simulink model "simF16_u04"  (R2023b)
settings: Solver=ode4  StartTime=0  StopTime=5  FixedStep=0.005  RelTol=1e-3  EnableMultiTasking=on
values from neighbouring files (symbols this model uses):
  control_trim = u0    [find_trim.m]    (also in trimcond.mat = [0.154059600013 -0.694715670316 -3.42749873112e-15 4.5481145; trimcond2.mat = [0.154007747083 -0.694801754663 0.00182544197392 0.000329744)
  state_trim = constraint( state )    [find_trim.m]    (also in trimcond.mat = [502 0.0505701217863 2.65111802467e-16 0 0.0505701217863 0 0; trimcond2.mat = [501.999976668 0.0505473192089 -2.30406790676e-05 0.00010278)
settings Model: Creator=keviczky  LastModifiedBy=suvo
settings DataIOCC: Decimation=50  SaveFormat=Array  SignalLoggingSaveFormat=ModelDataLogs  ReturnWorkspaceOutputs=off  SignalLoggingName=sigsOut
settings OptimizationCC: BooleanDataType=off
settings DebuggingCC: SaveWithParameterizedLinksMsg=none  UnderspecifiedInitializationDetection=Classic  MergeDetectMultiDrivingBlocksExec=none  SignalResolutionControl=TryResolveAllWithWarning  MultiTaskDSMMsg=warning  MultiTaskCondExecSysMsg=none  UnconnectedInputMsg=warning  UnconnectedOutputMsg=warning  UnconnectedLineMsg=warning
settings HardwareCC: ProdBitPerPointer=32  ProdBitPerSizeT=32  ProdBitPerPtrDiffT=32  ProdLargestAtomicFloat=None  ProdIntDivRoundTo=Undefined  ProdEndianess=Unspecified  ProdWordSize=32  ProdHWDeviceType=32-bit Generic  TargetUnknown=on
settings ModelReferenceCC: PropagateSignalLabelsOutOfModel=off
settings GRTTargetCC: CombineOutputUpdateFcns=off  GRTInterface=on
settings ConfigComp: CovMetricSettings=dw  CovSaveCumulativeToWorkspaceVar=on  CovSaveSingleToWorkspaceVar=on

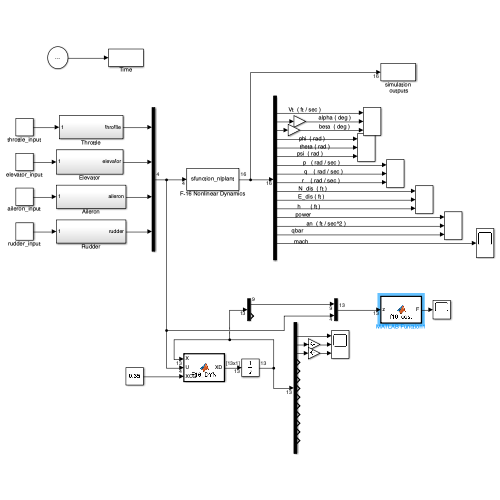
[thumbnail: Simulink's stored preview of the top-level diagram]
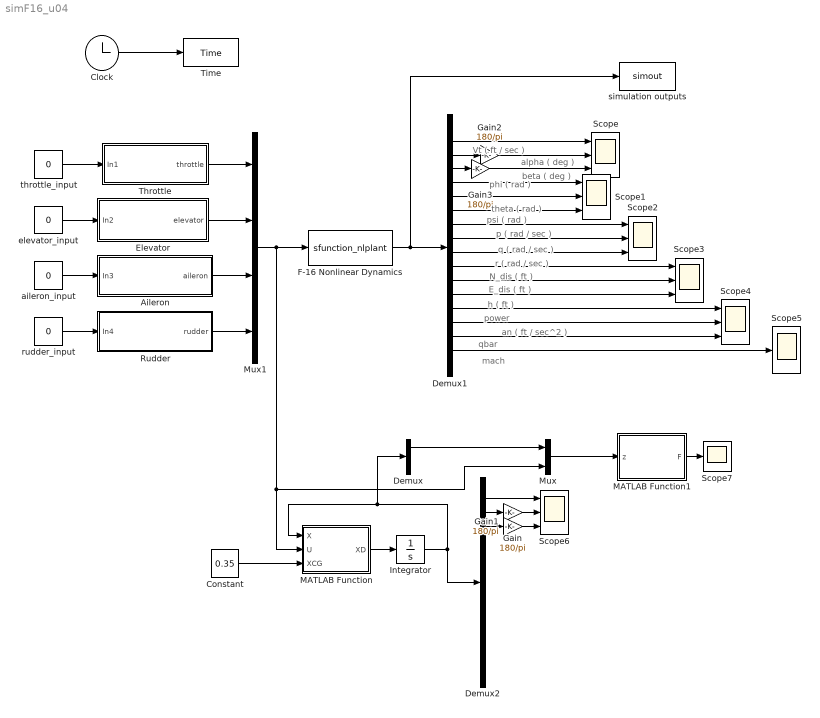
== system simF16_u04 ==
  note: Vt ( ft / sec )
  note: alpha ( deg )
  note: beta ( deg )
  note: phi ( rad )
  note: theta ( rad )
  note: psi ( rad )
  note: p ( rad / sec )
  note: q ( rad / sec )
  note: r ( rad / sec )
  note: N_dis ( ft )
  note: E_dis ( ft )
  note: h ( ft )
  note: power
  note: an ( ft / sec^2 )
  note: qbar
  note: mach
  Aileron : Subsystem
  Clock : Clock
      settings: Decimation=50
  Constant : Constant  Value=0.35
  Demux : Demux  Outputs=[9 4]
  Demux1 : Demux  Outputs=16
  Demux2 : Demux  Outputs=13
  Elevator : Subsystem
  F-16 Nonlinear Dynamics : S-Function  FunctionName=sfunction_nlplant  Parameters="state_trim,  xcg"  SFunctionDeploymentMode=off  EnableBusSupport=off
  Gain{,1..3} (4 alike) : Gain  Gain=180/pi
  Integrator : Integrator  InitialCondition=[state_trim]
  MATLAB Function : MATLAB Function  TreatAsAtomicUnit=on
  MATLAB Function1 : MATLAB Function  TreatAsAtomicUnit=on
  Mux : Mux  Inputs=2
  Mux1 : Mux
  Rudder : Subsystem
  Scope{,1..4,6} (6 alike) : Scope  NumInputPorts=3
  Scope5 : Scope
  Scope7 : Scope
  Throttle : Subsystem
  Time : ToWorkspace  VariableName=Time  SampleTime=-1
      settings: Decimation=100
  aileron_input : Constant  Value=0
  elevator_input : Constant  Value=0
  rudder_input : Constant  Value=0
  simulation outputs : ToWorkspace  VariableName=simout  SampleTime=-1
      settings: Decimation=100
  throttle_input : Constant  Value=0
  wires:
  F-16 Nonlinear Dynamics/1 -> Demux1/1, simulation outputs/1
  Clock/1 -> Time/1
  Demux1/1 -> Scope/1
  Demux1/2 -> Gain2/1
  Demux1/3 -> Gain3/1
  Demux1/5 -> Scope1/2
  Demux1/6 -> Scope1/3
  Demux1/7 -> Scope2/1
  Demux1/8 -> Scope2/2
  Demux1/9 -> Scope2/3
  Demux1/10 -> Scope3/1
  Demux1/11 -> Scope3/2
  Demux1/12 -> Scope3/3
  Demux1/13 -> Scope4/1
  Demux1/14 -> Scope4/2
  Demux1/4 -> Scope1/1
  Demux1/15 -> Scope4/3
  Demux1/16 -> Scope5/1
  Throttle/1(throttle) -> Mux1/1
  Elevator/1(elevator) -> Mux1/2
  Aileron/1(aileron) -> Mux1/3
  Rudder/1(rudder) -> Mux1/4
  throttle_input/1 -> Throttle/1(In1)
  elevator_input/1 -> Elevator/1(In2)
  aileron_input/1 -> Aileron/1(In3)
  rudder_input/1 -> Rudder/1(In4)
  MATLAB Function/1(XD) -> Integrator/1
  Integrator/1 -> Demux2/1, Demux/1, MATLAB Function/1(X)
  Mux1/1 -> MATLAB Function/2(U), Mux/2, F-16 Nonlinear Dynamics/1
  Demux2/1 -> Scope6/1
  Demux2/2 -> Gain/1
  Demux2/3 -> Gain1/1
  Constant/1 -> MATLAB Function/3(XCG)
  Gain/1 -> Scope6/2
  Gain1/1 -> Scope6/3
  Gain2/1 -> Scope/2
  Gain3/1 -> Scope/3
  MATLAB Function1/1(F) -> Scope7/1
  Demux/1 -> Mux/1
  Mux/1 -> MATLAB Function1/1(z)

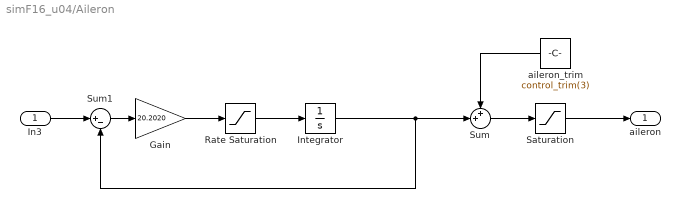
== system simF16_u04/Aileron ==
  In3 : Inport
  Gain : Gain  Gain=20.2020  SaturateOnIntegerOverflow=on  OutDataTypeStr=Inherit: Same as input  ParamDataTypeStr=Inherit: Same as input
  Integrator : Integrator  UpperSaturationLimit=21.5  LowerSaturationLimit=-21.5
  Rate Saturation : Saturate  UpperLimit=80  LowerLimit=-80
  Saturation : Saturate  UpperLimit=21.5  LowerLimit=-21.5
  Sum : Sum  Inputs=++|  InputSameDT=on  SaturateOnIntegerOverflow=on  OutDataTypeStr=Inherit: Same as first input
  Sum1 : Sum  Inputs=|+-  InputSameDT=on  SaturateOnIntegerOverflow=on  OutDataTypeStr=Inherit: Same as first input
  aileron_trim : Constant  Value=control_trim(3)
  aileron : Outport
  wires:
  In3/1 -> Sum1/1
  Sum1/1 -> Gain/1
  Gain/1 -> Rate Saturation/1
  Rate Saturation/1 -> Integrator/1
  Integrator/1 -> Sum1/2, Sum/2
  Sum/1 -> Saturation/1
  aileron_trim/1 -> Sum/1
  Saturation/1 -> aileron/1

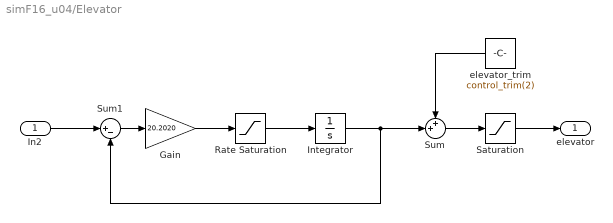
== system simF16_u04/Elevator ==
  In2 : Inport
  Gain : Gain  Gain=20.2020  SaturateOnIntegerOverflow=on  OutDataTypeStr=Inherit: Same as input  ParamDataTypeStr=Inherit: Same as input
  Integrator : Integrator  UpperSaturationLimit=25  LowerSaturationLimit=-25
  Rate Saturation : Saturate  UpperLimit=60  LowerLimit=-60
  Saturation : Saturate  UpperLimit=25  LowerLimit=-25
  Sum : Sum  Inputs=++|  InputSameDT=on  SaturateOnIntegerOverflow=on  OutDataTypeStr=Inherit: Same as first input
  Sum1 : Sum  Inputs=|+-  InputSameDT=on  SaturateOnIntegerOverflow=on  OutDataTypeStr=Inherit: Same as first input
  elevator_trim : Constant  Value=control_trim(2)
  elevator : Outport
  wires:
  In2/1 -> Sum1/1
  Sum1/1 -> Gain/1
  Gain/1 -> Rate Saturation/1
  Rate Saturation/1 -> Integrator/1
  Integrator/1 -> Sum1/2, Sum/2
  Sum/1 -> Saturation/1
  elevator_trim/1 -> Sum/1
  Saturation/1 -> elevator/1

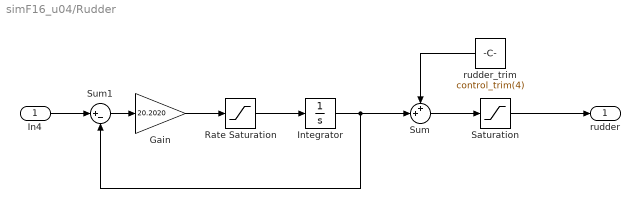
== system simF16_u04/Rudder ==
  In4 : Inport
  Gain : Gain  Gain=20.2020  SaturateOnIntegerOverflow=on  OutDataTypeStr=Inherit: Same as input  ParamDataTypeStr=Inherit: Same as input
  Integrator : Integrator  UpperSaturationLimit=30  LowerSaturationLimit=-30
  Rate Saturation : Saturate  UpperLimit=120  LowerLimit=-120
  Saturation : Saturate  UpperLimit=30  LowerLimit=-30
  Sum : Sum  Inputs=++|  InputSameDT=on  SaturateOnIntegerOverflow=on  OutDataTypeStr=Inherit: Same as first input
  Sum1 : Sum  Inputs=|+-  InputSameDT=on  SaturateOnIntegerOverflow=on  OutDataTypeStr=Inherit: Same as first input
  rudder_trim : Constant  Value=control_trim(4)
  rudder : Outport
  wires:
  In4/1 -> Sum1/1
  Sum1/1 -> Gain/1
  Gain/1 -> Rate Saturation/1
  Rate Saturation/1 -> Integrator/1
  Integrator/1 -> Sum1/2, Sum/2
  Saturation/1 -> rudder/1
  Sum/1 -> Saturation/1
  rudder_trim/1 -> Sum/1

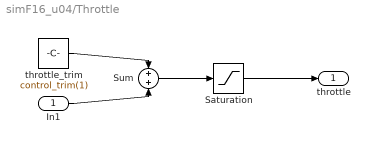
== system simF16_u04/Throttle ==
  In1 : Inport
  Saturation : Saturate  UpperLimit=1  LowerLimit=0
  Sum : Sum  InputSameDT=on  SaturateOnIntegerOverflow=on  OutDataTypeStr=Inherit: Same as first input
  throttle_trim : Constant  Value=control_trim(1)
  throttle : Outport
  wires:
  throttle_trim/1 -> Sum/1
  In1/1 -> Sum/2
  Sum/1 -> Saturation/1
  Saturation/1 -> throttle/1

== matlab function simF16_u04/MATLAB Function ==
  data: X input; U input; XD output; XCG input
function XD = F16_DYN(X,U,XCG)
% f16 dynamics

% Author: Subhabrata Ganguli
%
% Ref: Stevens, Brian L.; Lewis, Frank L.; Johnson, Eric N.. 
% Aircraft Control and Simulation: Dynamics, 
% Controls Design, and Autonomous Systems. 
% Wiley.

%% Parameters

AXX = 9496.0;
AYY = 55814.0;
AZZ = 63100.0;
AXZ =   982.0;

AXZS = AXZ^2;
XPQ  = AXZ * (AXX - AYY + AZZ);
GAM = AXX * AZZ - AXZ^2;

XQR = AZZ * (AZZ - AYY) + AXZS;
ZPQ =(AXX-AYY) * AXX + AXZS;
YPR = AZZ - AXX;

WEIGHT = 25000.0;
GD = 32.174;
MASS = WEIGHT/GD;
%MASS = 636.942675159236;

S = 300;
B = 30;
CBAR = 11.32;
XCGR = 0.35;
HX = 160;
RTOD = 180/pi;

%% Assign State and Control Variables

VT = X(1); 
ALPHA = X(2)*RTOD; 
BETA = X(3)*RTOD;
PHI = X(4); 
THETA = X(5); 
PSI = X(6);
P = X(7); 
Q = X(8); 
R = X(9); 
ALT = X(12); 
POW = X(13);

THTL = U(1);
EL = U(2);
AIL = U(3);
RDR = U(4);

XD = zeros(13,1);

%% Air data computer and engine model

[TFAC, T, RHO, AMACH, QBAR, PS ] = ADC (VT, ALT);
CPOW = TGEAR(THTL);

XD(13) = PDOT(POW,CPOW);     
T = THRUST(POW,ALT,AMACH);

%% Look-up tables and component buildup

CXT = CX (ALPHA,EL);
CYT = CY (BETA,AIL,RDR);
CZT = CZ (ALPHA,BETA,EL);
      
DAIL= AIL/20.0; DRDR= RDR/30.0;

DLDA_OUT = DLDA(ALPHA,BETA);
DLDR_OUT = DLDR(ALPHA,BETA);
DNDA_OUT = DNDA(ALPHA,BETA);
DNDR_OUT = DNDR(ALPHA,BETA);

CLT = CL(ALPHA,BETA) + DLDA_OUT*DAIL + DLDR_OUT*DRDR;
CMT = CM(ALPHA,EL);
CNT = CN(ALPHA,BETA) + DNDA_OUT*DAIL + DNDR_OUT*DRDR;

%% Add damping derivatives

TVT = 0.5/VT; 
B2V = B*TVT; 
CQ = CBAR*Q*TVT;

D = DAMP(ALPHA);

CXT = CXT + CQ * D(1);
CYT = CYT + B2V * ( D(2)*R + D(3)*P );
CZT = CZT + CQ * D(4);
CLT = CLT + B2V * ( D(5)*R + D(6)*P );
CMT = CMT + CQ * D(7) + CZT * (XCGR-XCG);
CNT = CNT + B2V*(D(8)*R + D(9)*P) - CYT*(XCGR-XCG) * CBAR/B;

%% Get ready for state equations

CBTA  = cos(X(3)); 
U     = VT*cos(X(2))*CBTA;
V     = VT * sin(X(3)); 
W     = VT*sin(X(2))*CBTA;
STH   = sin(THETA); 
CTH   = cos(THETA);   
SPH   = sin(PHI);
CPH   = cos(PHI); 
SPSI  = sin(PSI);    
CPSI  = cos(PSI);
QS    = QBAR * S; 
QSB   = QS * B;        
RMQS  = QS/MASS;
GCTH  = GD * CTH; 
QSPH  = Q * SPH;
AY    = RMQS*CYT; 
AZ    = RMQS * CZT;

%% Force Equations

UDOT   = R*V - Q*W - GD*STH + (QS * CXT + T)/MASS;
VDOT   = P*W - R*U + GCTH * SPH + AY;
WDOT   = Q*U - P*V + GCTH * CPH + AZ;
    
DUM   = (U*U + W*W);
XD(1) = (U*UDOT + V*VDOT + W*WDOT)/VT;
XD(2) = (U*WDOT - W*UDOT) / DUM;
XD(3) = (VT*VDOT- V*XD(1)) * CBTA / DUM;

%% Kinematics

XD(4) = P + (STH/CTH)*(QSPH + R*CPH);
XD(5) = Q*CPH - R*SPH;
XD(6) = (QSPH + R*CPH)/CTH;

%% Moments

ROLL  = QSB*CLT;
PITCH = QS *CBAR*CMT;
YAW   = QSB*CNT;
PQ    = P*Q;
QR    = P*R;
QHX   = Q*HX;
XD(7) = ( XPQ*PQ - XQR*QR + AZZ*ROLL + AXZ*(YAW + QHX) )/GAM;
XD(8) = ( YPR*P*R - AXZ*(P^2 - R^2) + PITCH - R*HX )/AYY;
XD(9) = ( ZPQ*PQ - XPQ*QR + AXZ*ROLL + AXX*(YAW + QHX) )/GAM;

%% Navigation

T1 = SPH * CPSI; 
T2 = CPH * STH; 
T3 = SPH * SPSI;
S1 = CTH * CPSI; 
S2 = CTH * SPSI; 
S3 = T1 * STH - CPH * SPSI;
S4 = T3 * STH + CPH * CPSI; 
S5 = SPH * CTH; 
S6 = T2 * CPSI + T3;
S7 = T2 * SPSI - T1; 
S8 = CPH * CTH;

XD(10)  = U * S1 + V * S3 + W * S6;   %   North speed
XD(11)  = U * S2 + V * S4 + W * S7;   %   East speed
XD(12)  = U * STH -V * S5 - W * S8;   %   Vertical speed

XD = XD(:);

end

== matlab function simF16_u04/MATLAB Function1 ==
  data: z input; F output
function F = f16_cost(z)

x = zeros(13,1);
x(1:9) = z(1:9);

u = z(10:13);

x(13) = TGEAR(u(1));

xdot = F16_DYN(x,u,0.35);
V = x(1);
alpha = x(2);
theta = x(5);
gam = theta - alpha;
beta = x(3);
phi = x(4);
psi = x(6);
pqr = x(7:9);

Q = [xdot(1:9);
     V - 502;
     gam;
     beta;
     phi;
     psi;
     pqr;
    ];

H = eye(17)*1e3;

%H([2 3 7 8 9]) = 100*H([2 3 7 8 9]);

F = Q'*H*Q;

% XD(1)**2 + 100.0*( XD(2)**2 + XD(3)**2 )
% &      + 10.0*( XD(7)**2 + XD(8)**2 + XD(9)**2 )


end
